simulink model "fskdoc"  (Simulink 6.0)
settings: Solver=ode45  SolverMode=SingleTasking  StartTime=0.0  StopTime=15  RelTol=1e-3
undefined symbols (not defined in the file or in its folder): slcm
libraries: commdigbbndfm2 x2, commchan2 x1, commrandsrc2 x1, dspsigops x1, commsink2 x1
settings Model: Creator=ptrow  LastModifiedBy=agaltman  ProdHWDeviceType=Specified
settings DataIOCC: SaveOutput=off  SaveTime=off  SignalLoggingName=sigsOut
settings OptimizationCC: BooleanDataType=off  InlineParams=on  MultiInstanced=off
settings FormatCC: IgnoreBidirectionalLines=off
settings DebuggingCC: AlgebraicLoopMsg=error
settings HardwareCC: ProdHWDeviceType=Specified
settings CodeAppCC: FileBanners=off  CustomSymbols=off  MangleLength=5
settings GRTTargetCC: TargetFcnLib=iso_c_tmw.mat  IsERTTarget=off

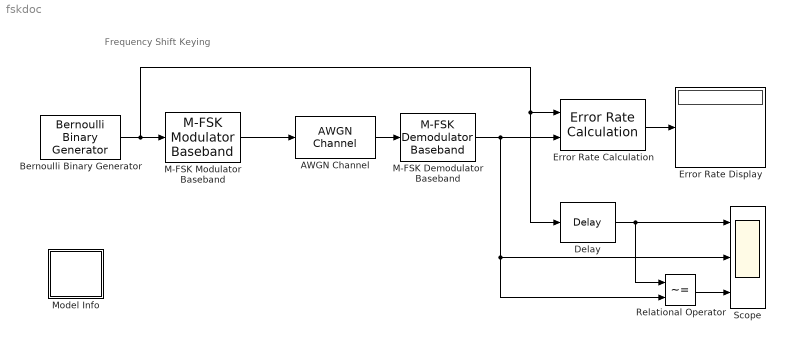
== system fskdoc ==
  note: Frequency Shift Keying
  AWGN Channel : commchan2/AWGN Channel  seed=113  noiseMode="Signal to noise ratio  (Es/No)"  EbNodB=10  EsNodB=10  SNRdB=10  bitsPerSym=1  Ps=1  Tsym=1/1200  variance=1
  Bernoulli Binary Generator : commrandsrc2/Bernoulli Binary Generator  P=0.5  seed=89  Ts=1/1200  frameBased=off  sampPerFrame=1  orient=off
  Delay : dspsigops/Delay  dly_unit=Samples  delay=1  ic_detail=off  dif_ic_for_ch=off  dif_ic_for_dly=off  ic=0  reset_popup=None
  Error Rate Calculation : commsink2/Error Rate Calculation  N=1  st_delay=0  cp_mode=Entire frame  subframe=[]  PMode=Port  WsName=ErrorVec  RsMode2=off  stop=off  numErr=100  maxBits=1e5
  Error Rate Display : Display
  M-FSK Demodulator Baseband : commdigbbndfm2/M-FSK Demodulator Baseband  M=2  OutType=Integer  Dec=Binary  freqSep=1000  numSamp=5
  M-FSK Modulator Baseband : commdigbbndfm2/M-FSK Modulator Baseband  M=2  InType=Integer  Enc=Binary  freqSep=1000  phaseType=Continuous  numSamp=5
  Model Info : Subsystem  LoadFcn=slcm LoadBlock;  InitFcn=slcm('UpdateAllCMBlocksInThisModelInit')  mask(CMBlock){InitialSaveTempField=, InitialBlockCM=None, BlockCM=None, Frame=on, SaveTempField=, DisplayStringWithTags=Info, MaskDisplayString=Info, HorizontalTextAlignment=Center, LeftAlignmentValue=0.5, SourceBlockDiagram=fskdoc, TagMaxNumber=20, CMTag1=, CMTag2=, CMTag3=, CMTag4=, CMTag5=, CMTag6=, CMTag7=, CMTag8=, CMTag9=, CMTag10=, CMTag11=, CMTag12=, CMTag13=, CMTag14=, CMTag15=, CMTag16=, CMTag17=, CMTag18=, CMTag19=, CMTag20=}
      mask help: This block allows revision control information to be displayed within the model.
      settings: CopyFcn=slcm CopyBlock;  DeleteFcn=slcm Cancel;  PostSaveFcn=slcm('UpdateAllCMBlocksInThisModel')  NameChangeFcn=slcm Rename;  OpenFcn=commdemohelp;
      mask Display: text(str2num(LeftAlignmentValue), 0.5, MaskDisplayString, 'HorizontalAlignment', HorizontalTextAlignment)
  Relational Operator : RelationalOperator  Operator=~=  InputSameDT=on
  Scope : Scope  NumInputPorts=3
      settings: TimeRange=1  YMin=-1~-1~-1  YMax=2~2~2
  wires:
  M-FSK Demodulator Baseband/1 -> Scope/2, Relational Operator/2, Error Rate Calculation/2
  M-FSK Modulator Baseband/1 -> AWGN Channel/1
  AWGN Channel/1 -> M-FSK Demodulator Baseband/1
  Delay/1 -> Relational Operator/1, Scope/1
  Bernoulli Binary Generator/1 -> Error Rate Calculation/1, Delay/1, M-FSK Modulator Baseband/1
  Error Rate Calculation/1 -> Error Rate Display/1
  Relational Operator/1 -> Scope/3

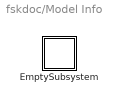
== system fskdoc/Model Info ==
  EmptySubsystem : Subsystem

== system fskdoc/Model Info/EmptySubsystem ==
